simulink model "Micro_mouse"  (R2024b)
settings: Solver=FixedStepAuto  StartTime=0.0  StopTime=inf  FixedStep=0.01  RelTol=1e-3  EnableMultiTasking=on
undefined symbols (not defined in the file): DiscIntNeverNeededParam
libraries: stm32f4xxblockslib x7, simulink x4, stm32l4xxblockslib x4, slpidlib x2
settings Model: STM32="{\"PWMOutput\":[{\"ID\":\"untitled1:1\"},{\"ID\":\"Micro_mouse:1\"},{\"ID\":\"Micro_mouse:135\"},{\"ID\":\"Micro_mouse:163\"}],\"DigitalPortWrite\":[{\"ID\":\"untitled1:2\"},{\"ID\":\"Micro_mouse:2\"},{\"ID\":\"Micro_mouse:133\"},{\"ID\":\"Micro_mouse:161\"}],\"AnalogInput\":{\"ID\":\"Micro_mouse:28\"},\"DigitalPortRead\":[{\"ID\":\"Micro_mouse:101\"},{\"ID\":\"Micro_mouse:116\"},{\"ID\":\"Micro_mouse:141\"},{\"ID\":\"Micro_mouse:142\"},{\"ID\":\"Micro_mouse:169\"},{\"ID\":\"Micro_mouse:170\"}],\"HardwareInterrupt\":[{\"ID\":\"Micro_mouse:132\"},{\"ID\":\"Micro_mouse:160\"}]}"  Creator=galgi  LastModifiedBy=galgi
settings SolverCC: AutoInsertRateTranBlk=on
settings OptimizationCC: DefaultParameterBehavior=Inlined  EnhancedBackFolding=on  PassReuseOutputArgsAs=Individual arguments  ZeroExternalMemoryAtStartup=off  ZeroInternalMemoryAtStartup=off  MaxStackSize=512  OptimizeBlockOrder=speed  DifferentSizesBufferReuse=on  EfficientTunableParamExpr=on
settings DebuggingCC: ParameterTunabilityLossMsg=error
settings HardwareCC: ProdBitPerPointer=32  ProdBitPerSizeT=32  ProdBitPerPtrDiffT=32  ProdLargestAtomicInteger=Long  ProdLargestAtomicFloat=Double  ProdWordSize=32  ProdLongLongMode=on  ProdHWDeviceType=ARM Compatible->ARM Cortex-M
settings SFSimCC: MATLABDynamicMemAlloc=off
settings RTWCC: Description=Embedded Coder  SystemTargetFile=ert.tlc  HardwareBoard=STM32L4xx Based  TemplateMakefile=ert_default_tmf  Toolchain=GNU Tools for ARM Embedded Processors
settings CodeAppCC: ForceParamTrailComments=on  IgnoreCustomStorageClasses=off  OperatorAnnotations=on  SimulinkDataObjDesc=on  SFDataObjDesc=on  InsertBlockDesc=on
settings ERTTargetCC: TargetLangStandard=C99 (ISO)  CodeReplacementLibrary=ARM Cortex-M  SupportContinuousTime=on  ExtModeTransport=3  ExtModeStaticAlloc=on  ExtModeStaticAllocSize=2048  ExtModeMexFile=ext_xcp  ExtModeIntrfLevel=Level2 - Open

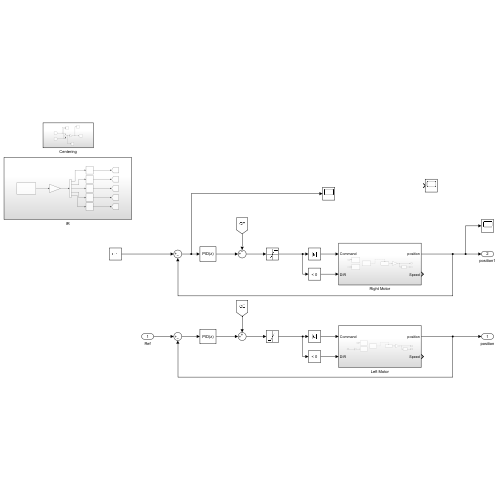
[thumbnail: Simulink's stored preview of the top-level diagram]
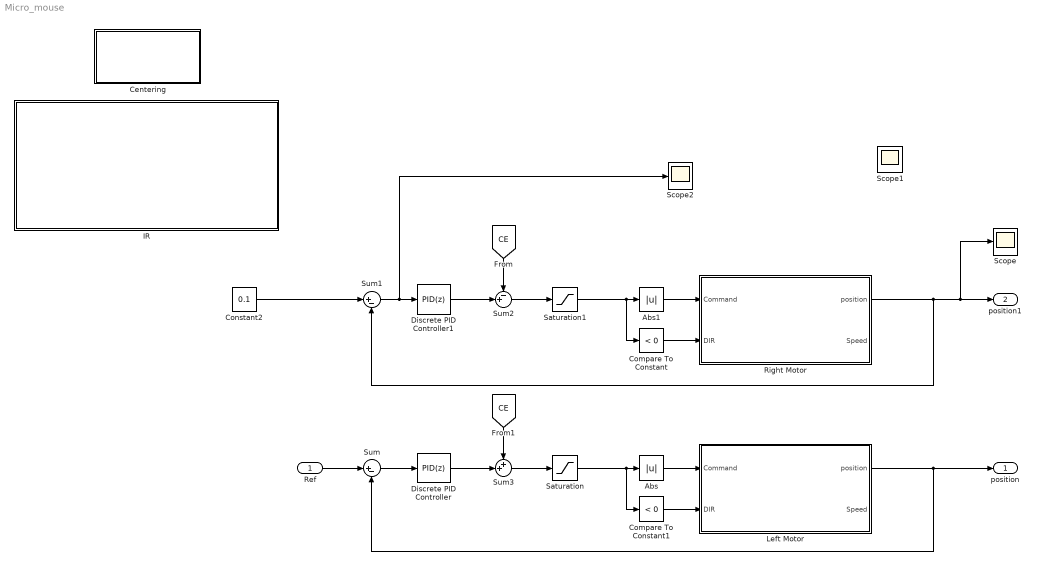
== system Micro_mouse ==
  Ref : Inport
  Abs : Abs  SaturateOnIntegerOverflow=off
  Abs1 : Abs  SaturateOnIntegerOverflow=off
  Centering : Subsystem
  Compare To Constant : simulink/Logic and Bit Operations/Compare To Constant  relop=<  const=0  OutDataTypeStr=boolean
  Compare To Constant1 : simulink/Logic and Bit Operations/Compare To Constant  relop=<  const=0  OutDataTypeStr=boolean
  Constant2 : Constant  Value=0.1
  Discrete PID Controller : slpidlib/PID Controller  Controller=PID  Form=Parallel  TimeDomain=Discrete-time  UseExternalTs=off  SampleTime=-1  IntegratorMethod=Forward Euler  FilterMethod=Forward Euler  ControllerParametersSource=internal  P=1  I=1  UseKiTs=off  D=0  UseExternalDerivativeSource=off  N=100  UseFilter=on  TunerSelectOption=Transfer Function Based (PID Tuner App)  InitialConditionSource=internal  InitialConditionForIntegrator=0  InitialConditionForFilter=0  DifferentiatorICPrevScaledInput=0  ExternalReset=none  TrackingMode=off  Kt=1  LimitOutput=off  SatLimitsSource=internal  UpperSaturationLimit=inf  LowerSaturationLimit=-inf  LinearizeAsGain=off  AntiWindupMode=none  Kb=1  LimitIntegrator=off  UpperIntegratorSaturationLimit=inf  LowerIntegratorSaturationLimit=-inf  POutMin=[]  POutMax=[]  IOutMin=[]  IOutMax=[]  DOutMin=[]  DOutMax=[]  NOutMin=[]  NOutMax=[]  SumOutMin=[]  SumOutMax=[]  SaturationOutMin=[]  SaturationOutMax=[]  PParamMin=[]  PParamMax=[]  IParamMin=[]  IParamMax=[]  DParamMin=[]  DParamMax=[]  NParamMin=[]  NParamMax=[]  KbParamMin=[]  KbParamMax=[]  KtParamMin=[]  KtParamMax=[]  KbOutMin=[]  KbOutMax=[]  KtOutMin=[]  KtOutMax=[]  IntegratorOutMin=[]  IntegratorOutMax=[]  FilterOutMin=[]  FilterOutMax=[]  SumI1OutMin=[]  SumI1OutMax=[]  SumI2OutMin=[]  SumI2OutMax=[]  SumI3OutMin=[]  SumI3OutMax=[]  SumI4OutMin=[]  SumI4OutMax=[]  SumDOutMin=[]  SumDOutMax=[]  DifferentiatorOutMin=[]  DifferentiatorOutMax=[]  FilterDiffOutCoefMin=[]  FilterDiffOutCoefMax=[]  ReciprocalOutMin=[]  ReciprocalOutMax=[]  SumDenOutMin=[]  SumDenOutMax=[]  SumNumOutMin=[]  SumNumOutMax=[]  DivideOutMin=[]  DivideOutMax=[]  UdiffTsProdOutMin=[]  UdiffTsProdOutMax=[]  NTsProdOutMin=[]  NTsProdOutMax=[]  UintegralTsProdOutMin=[]  UintegralTsProdOutMax=[]  UngainTsProdOutMin=[]  UngainTsProdOutMax=[]  ClampingZeroOutDataTypeStr=Inherit: Inherit via back propagation  ClampingZeroOutMin=[]  ClampingZeroOutMax=[]  FilterDenConstantOutDataTypeStr=Inherit: Inherit via back propagation  FilterDenConstantOutMin=[]  FilterDenConstantOutMax=[]  PCopyOutDataTypeStr=Inherit: Inherit via back propagation  PCopyOutMin=[]  PCopyOutMax=[]  NCopyOutDataTypeStr=Inherit: Inherit via back propagation  NCopyOutMin=[]  NCopyOutMax=[]  IntegratorContinuousStateAttributes=''  IntegratorStateMustResolveToSignalObject=off  IntegratorRTWStateStorageClass=Auto  FilterContinuousStateAttributes=''  FilterStateMustResolveToSignalObject=off  FilterRTWStateStorageClass=Auto  ParallelPVariant=InternalParameters  IdealPVariant=Disabled  IVariant=InternalParameters  DVariant=InternalParameters  IntegratorVariant=Discrete  SatVariant=Disabled  AWVariant=Passthrough  PCopyVariant=Disabled  TRVariant=Disabled  FdbkBlocksVariant=Forward  IdealPFdbkVariant=Disabled  SatFdbkVariant=Disabled  DerivativeFilterVariant=ForwardEulerFilter  NVariant=InternalParameters  NCopyVariant=Disabled  FilterICVariant=InternalICsFilter  IntegratorICVariant=InternalICs  ExternalResetVariant=Disabled  TRSumVariant=Passthrough  SumFdbkVariant=Disabled  SumVariant=Sum_PID  TsampFilterVariant=InternalTs  TsampNgainVariant=Passthrough  TsampIntegralVariant=Disabled_SignalSpec  ExternalSaturationOutDataTypeStr=Inherit: Same as second input  DerivativeSourceVariant=ErrorSignal  PreIntVariant=InternalPreInt
      settings: LibrarySourceBlock=simulink/Discrete/Discrete PID Controller
  Discrete PID Controller1 : slpidlib/PID Controller  Controller=PID  Form=Parallel  TimeDomain=Discrete-time  UseExternalTs=off  SampleTime=-1  IntegratorMethod=Forward Euler  FilterMethod=Forward Euler  ControllerParametersSource=internal  P=1  I=1  UseKiTs=off  D=0  UseExternalDerivativeSource=off  N=100  UseFilter=on  TunerSelectOption=Transfer Function Based (PID Tuner App)  InitialConditionSource=internal  InitialConditionForIntegrator=0  InitialConditionForFilter=0  DifferentiatorICPrevScaledInput=0  ExternalReset=none  TrackingMode=off  Kt=1  LimitOutput=off  SatLimitsSource=internal  UpperSaturationLimit=inf  LowerSaturationLimit=-inf  LinearizeAsGain=off  AntiWindupMode=none  Kb=1  LimitIntegrator=off  UpperIntegratorSaturationLimit=inf  LowerIntegratorSaturationLimit=-inf  POutMin=[]  POutMax=[]  IOutMin=[]  IOutMax=[]  DOutMin=[]  DOutMax=[]  NOutMin=[]  NOutMax=[]  SumOutMin=[]  SumOutMax=[]  SaturationOutMin=[]  SaturationOutMax=[]  PParamMin=[]  PParamMax=[]  IParamMin=[]  IParamMax=[]  DParamMin=[]  DParamMax=[]  NParamMin=[]  NParamMax=[]  KbParamMin=[]  KbParamMax=[]  KtParamMin=[]  KtParamMax=[]  KbOutMin=[]  KbOutMax=[]  KtOutMin=[]  KtOutMax=[]  IntegratorOutMin=[]  IntegratorOutMax=[]  FilterOutMin=[]  FilterOutMax=[]  SumI1OutMin=[]  SumI1OutMax=[]  SumI2OutMin=[]  SumI2OutMax=[]  SumI3OutMin=[]  SumI3OutMax=[]  SumI4OutMin=[]  SumI4OutMax=[]  SumDOutMin=[]  SumDOutMax=[]  DifferentiatorOutMin=[]  DifferentiatorOutMax=[]  FilterDiffOutCoefMin=[]  FilterDiffOutCoefMax=[]  ReciprocalOutMin=[]  ReciprocalOutMax=[]  SumDenOutMin=[]  SumDenOutMax=[]  SumNumOutMin=[]  SumNumOutMax=[]  DivideOutMin=[]  DivideOutMax=[]  UdiffTsProdOutMin=[]  UdiffTsProdOutMax=[]  NTsProdOutMin=[]  NTsProdOutMax=[]  UintegralTsProdOutMin=[]  UintegralTsProdOutMax=[]  UngainTsProdOutMin=[]  UngainTsProdOutMax=[]  ClampingZeroOutDataTypeStr=Inherit: Inherit via back propagation  ClampingZeroOutMin=[]  ClampingZeroOutMax=[]  FilterDenConstantOutDataTypeStr=Inherit: Inherit via back propagation  FilterDenConstantOutMin=[]  FilterDenConstantOutMax=[]  PCopyOutDataTypeStr=Inherit: Inherit via back propagation  PCopyOutMin=[]  PCopyOutMax=[]  NCopyOutDataTypeStr=Inherit: Inherit via back propagation  NCopyOutMin=[]  NCopyOutMax=[]  IntegratorContinuousStateAttributes=''  IntegratorStateMustResolveToSignalObject=off  IntegratorRTWStateStorageClass=Auto  FilterContinuousStateAttributes=''  FilterStateMustResolveToSignalObject=off  FilterRTWStateStorageClass=Auto  ParallelPVariant=InternalParameters  IdealPVariant=Disabled  IVariant=InternalParameters  DVariant=InternalParameters  IntegratorVariant=Discrete  SatVariant=Disabled  AWVariant=Passthrough  PCopyVariant=Disabled  TRVariant=Disabled  FdbkBlocksVariant=Forward  IdealPFdbkVariant=Disabled  SatFdbkVariant=Disabled  DerivativeFilterVariant=ForwardEulerFilter  NVariant=InternalParameters  NCopyVariant=Disabled  FilterICVariant=InternalICsFilter  IntegratorICVariant=InternalICs  ExternalResetVariant=Disabled  TRSumVariant=Passthrough  SumFdbkVariant=Disabled  SumVariant=Sum_PID  TsampFilterVariant=InternalTs  TsampNgainVariant=Passthrough  TsampIntegralVariant=Disabled_SignalSpec  ExternalSaturationOutDataTypeStr=Inherit: Same as second input  DerivativeSourceVariant=ErrorSignal  PreIntVariant=InternalPreInt
      settings: LibrarySourceBlock=simulink/Discrete/Discrete PID Controller
  IR : Subsystem
  Left Motor : Subsystem
  Right Motor : Subsystem
  Saturation : Saturate  UpperLimit=100  LowerLimit=0
  Saturation1 : Saturate  UpperLimit=100  LowerLimit=0
  Scope : Scope
  Scope1 : Scope
  Scope2 : Scope
  Sum : Sum  Inputs=|+-
  Sum1 : Sum  Inputs=|+-
  Sum2 : Sum  Inputs=-+|
  Sum3 : Sum  Inputs=++|
  position : Outport
  position1 : Outport  Port=2
  wires:
  Saturation/1 -> Compare To Constant1/1, Abs/1
  Ref/1 -> Sum/1
  Sum/1 -> Discrete PID Controller/1
  Left Motor/1(position) -> Sum/2, position/1
  Saturation1/1 -> Compare To Constant/1, Abs1/1
  Right Motor/1(position) -> Sum1/2, Scope/1, position1/1
  Sum1/1 -> Scope2/1, Discrete PID Controller1/1
  Discrete PID Controller1/1 -> Sum2/2
  Sum2/1 -> Saturation1/1
  [CE] -> Sum2/1
  [CE] -> Sum3/1
  Sum3/1 -> Saturation/1
  Discrete PID Controller/1 -> Sum3/2
  Compare To Constant/1 -> Right Motor/2(DIR)
  Compare To Constant1/1 -> Left Motor/2(DIR)
  Abs/1 -> Left Motor/1(Command)
  Abs1/1 -> Right Motor/1(Command)
  Constant2/1 -> Sum1/1

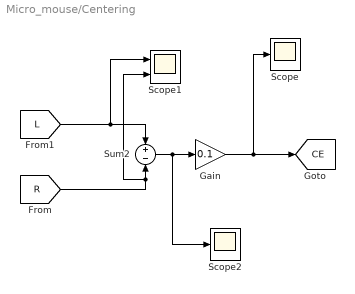
== system Micro_mouse/Centering ==
  Gain : Gain  Gain=0.1
  Scope : Scope
  Scope1 : Scope  NumInputPorts=2
  Scope2 : Scope
  Sum2 : Sum  Inputs=+|-
  tag scope: CE=global
  wires:
  [R] -> Scope1/2, Sum2/2
  [L] -> Scope1/1, Sum2/1
  Sum2/1 -> Scope2/1, Gain/1
  Gain/1 -> Scope/1, [CE]

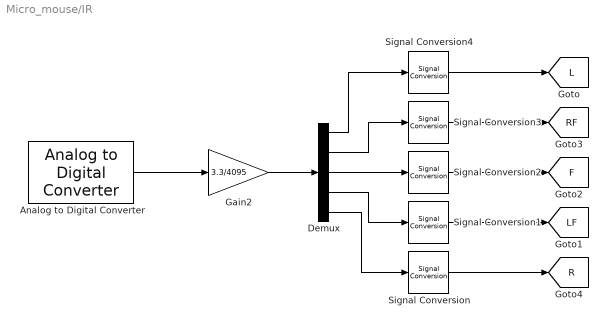
== system Micro_mouse/IR ==
  Analog to Digital Converter : stm32f4xxblockslib/Analog to Digital Converter  ADCModule=ADC1  ConversionGroup=Regular  TriggerMode=Trigger and read  NumberOfConversions=5  EnableBufferConv=off  BufferLength=1  OutputStatus=off  SampleTime=-1  EnableSimPort=off  hoistedMaskSrc=ECSoC/ECSimCodegen/Analog to Digital Converter
      settings: LibrarySourceBlock=stm32l4xxblockslib/Analog to Digital Converter
  Demux : Demux  Outputs=5
  Gain2 : Gain  Gain=3.3/4095
  Signal Conversion{,1..4} (5 alike) : SignalConversion  OverrideOpt=off
  tag scope: F=global, L=global, LF=global, R=global, RF=global
  wires:
  Demux/3 -> Signal Conversion2/1
  Demux/5 -> Signal Conversion/1
  Demux/4 -> Signal Conversion1/1
  Signal Conversion3/1 -> [RF]
  Analog to Digital Converter/1 -> Gain2/1
  Gain2/1 -> Demux/1
  Demux/2 -> Signal Conversion3/1
  Demux/1 -> Signal Conversion4/1
  Signal Conversion2/1 -> [F]
  Signal Conversion/1 -> [R]
  Signal Conversion1/1 -> [LF]
  Signal Conversion4/1 -> [L]

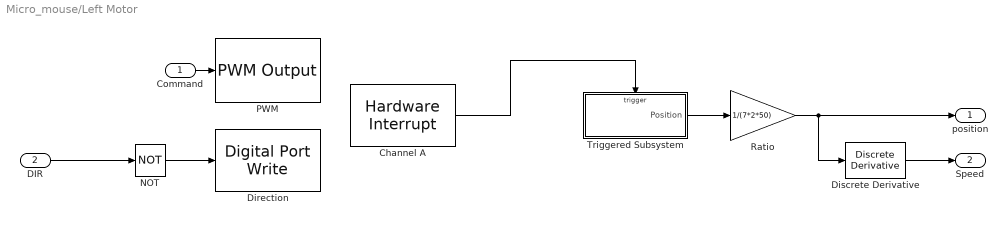
== system Micro_mouse/Left Motor ==
  Command : Inport
  DIR : Inport  Port=2
  Channel A : stm32l4xxblockslib/Hardware Interrupt  ISRGroup=External interrupts (EXTI)  ISRName=EXTI3_IRQHandler  ISRNumber=24  EventsList={ 'on', 'EXTI3 Event', '1'; 'off', 'Custom event', '2' }  SelectedEvents={'EXTI3 Event'}  TaskPriority=30  DisablePreemption=off  ClearInterruptFlagsAtEndOfEvent=off  InterruptDefinitionFile=$(TARGET_ROOT)/registry/interrupts/STM32F4xxBased_interrupts.xml  HardwareBoard=STM32L4xx Based  EnableSimPort=off
  Direction : stm32f4xxblockslib/Digital Port Write  PortName=GPIOA  PinNumber=[12]  ReadOperation=off  IOAsArray=on  EnableSimPort=off  hoistedMaskSrc=ECSoC/ECSimCodegen/Digital Port Write
      settings: LibrarySourceBlock=stm32l4xxblockslib/Digital Port Write
  Discrete Derivative : simulink/Discrete/Discrete Derivative  gainval=1.0  ICPrevScaledInput=0.0  OutMin=[]  OutMax=[]  OutDataType=fixdt(1, 16)  OutScaling=2^-10  DoSatur=off
  NOT : Logic  Operator=NOT  IconShape=distinctive  AllPortsSameDT=off
  PWM : stm32l4xxblockslib/PWM Output  TimerModule=TIM16  DutycycleUnits=Percentage  EnableChannel1=on  EnableChannel2=off  EnableChannel3=off  EnableChannel4=off  EnableChannel5=off  EnableChannel6=off  EnableCounterInput=off  EnableMainOutputInput=off  EnableFrequencyInput=off  SetRCAfterCE=off  OutputDirection=off  OutputMainOutputEnableStatus=off  SampleTime=0.1  EnableSimPort=off  EnableUpdateEvent=off  EnableCaptureCompare1Event=off  EnableCaptureCompare2Event=off  EnableCaptureCompare3Event=off  EnableCaptureCompare4Event=off  EnableTriggerEvent=off  EnableBreakEvent=off  EnableBreakEvent2=off  ProcessorFamily=STM32L4  hoistedMaskSrc=ECSoC/ECSimCodegen/PWM Output
  Ratio : Gain  Gain=1/(7*2*50)
  Triggered Subsystem : Subsystem  TreatAsAtomicUnit=on
  position : Outport
  Speed : Outport  Port=2
  wires:
  Command/1 -> PWM/1
  DIR/1 -> NOT/1
  Triggered Subsystem/1(Position) -> Ratio/1
  Channel A/1 -> Triggered Subsystem/Trigger
  Discrete Derivative/1 -> Speed/1
  Ratio/1 -> position/1, Discrete Derivative/1
  NOT/1 -> Direction/1

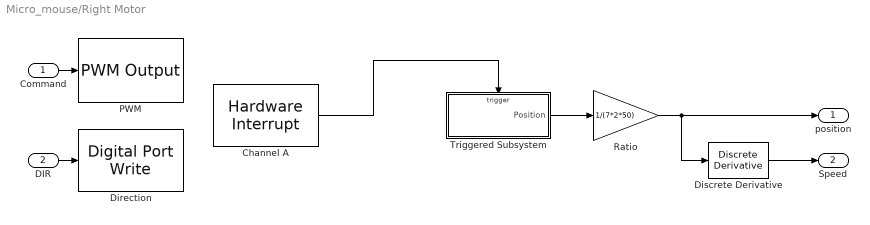
== system Micro_mouse/Right Motor ==
  Command : Inport
  DIR : Inport  Port=2
  Channel A : stm32l4xxblockslib/Hardware Interrupt  ISRGroup=External interrupts (EXTI)  ISRName=EXTI0_IRQHandler  ISRNumber=21  EventsList={ 'on', 'EXTI0 Event', '1'; 'off', 'Custom event', '2' }  SelectedEvents={'EXTI0 Event'}  TaskPriority=30  DisablePreemption=off  ClearInterruptFlagsAtEndOfEvent=off  InterruptDefinitionFile=$(TARGET_ROOT)/registry/interrupts/STM32F4xxBased_interrupts.xml  HardwareBoard=STM32L4xx Based  EnableSimPort=off
  Direction : stm32f4xxblockslib/Digital Port Write  PortName=GPIOA  PinNumber=[11]  ReadOperation=off  IOAsArray=on  EnableSimPort=off  hoistedMaskSrc=ECSoC/ECSimCodegen/Digital Port Write
      settings: LibrarySourceBlock=stm32l4xxblockslib/Digital Port Write
  Discrete Derivative : simulink/Discrete/Discrete Derivative  gainval=1.0  ICPrevScaledInput=0.0  OutMin=[]  OutMax=[]  OutDataType=fixdt(1, 16)  OutScaling=2^-10  DoSatur=off
  PWM : stm32l4xxblockslib/PWM Output  TimerModule=TIM1  DutycycleUnits=Percentage  EnableChannel1=on  EnableChannel2=off  EnableChannel3=off  EnableChannel4=off  EnableChannel5=off  EnableChannel6=off  EnableCounterInput=off  EnableMainOutputInput=off  EnableFrequencyInput=off  SetRCAfterCE=off  OutputDirection=off  OutputMainOutputEnableStatus=off  SampleTime=0.1  EnableSimPort=off  EnableUpdateEvent=off  EnableCaptureCompare1Event=off  EnableCaptureCompare2Event=off  EnableCaptureCompare3Event=off  EnableCaptureCompare4Event=off  EnableTriggerEvent=off  EnableBreakEvent=off  EnableBreakEvent2=off  ProcessorFamily=STM32L4  hoistedMaskSrc=ECSoC/ECSimCodegen/PWM Output
  Ratio : Gain  Gain=1/(7*2*50)
  Triggered Subsystem : Subsystem  TreatAsAtomicUnit=on
  position : Outport
  Speed : Outport  Port=2
  wires:
  Command/1 -> PWM/1
  DIR/1 -> Direction/1
  Triggered Subsystem/1(Position) -> Ratio/1
  Channel A/1 -> Triggered Subsystem/Trigger
  Discrete Derivative/1 -> Speed/1
  Ratio/1 -> position/1, Discrete Derivative/1

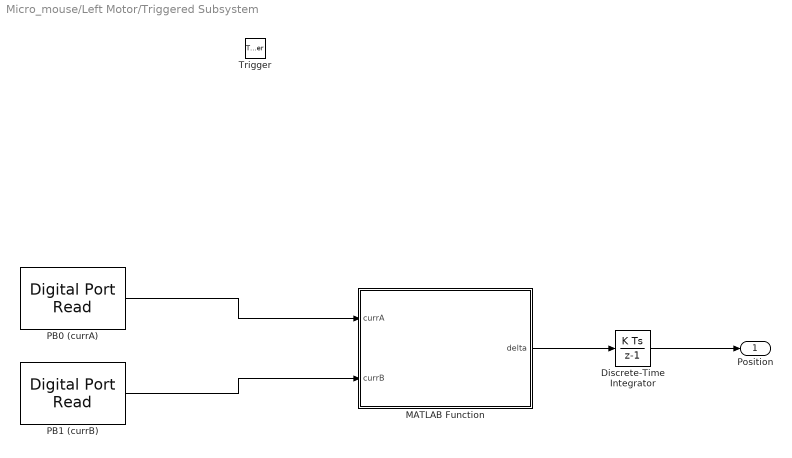
== system Micro_mouse/Left Motor/Triggered Subsystem ==
  Trigger : TriggerPort  TriggerType=function-call  VariantControl=(inherit)
  Discrete-Time Integrator : DiscreteIntegrator  SampleTime=-1  ICPrevOutput=DiscIntNeverNeededParam  ICPrevScaledInput=DiscIntNeverNeededParam
  MATLAB Function : MATLAB Function  TreatAsAtomicUnit=on
  PB0 (currA) : stm32f4xxblockslib/Digital Port Read  PortName=GPIOB  PinNumber=[3]  ReadOperation=on  IOAsArray=on  SampleTime=-1  EnableSimPort=off  hoistedMaskSrc=ECSoC/ECSimCodegen/Digital Port Read
      settings: LibrarySourceBlock=stm32l4xxblockslib/Digital Port Read
  PB1 (currB) : stm32f4xxblockslib/Digital Port Read  PortName=GPIOB  PinNumber=[4]  ReadOperation=on  IOAsArray=on  SampleTime=-1  EnableSimPort=off  hoistedMaskSrc=ECSoC/ECSimCodegen/Digital Port Read
      settings: LibrarySourceBlock=stm32l4xxblockslib/Digital Port Read
  Position : Outport
  wires:
  PB1 (currB)/1 -> MATLAB Function/2(currB)
  PB0 (currA)/1 -> MATLAB Function/1(currA)
  Discrete-Time Integrator/1 -> Position/1
  MATLAB Function/1(delta) -> Discrete-Time Integrator/1

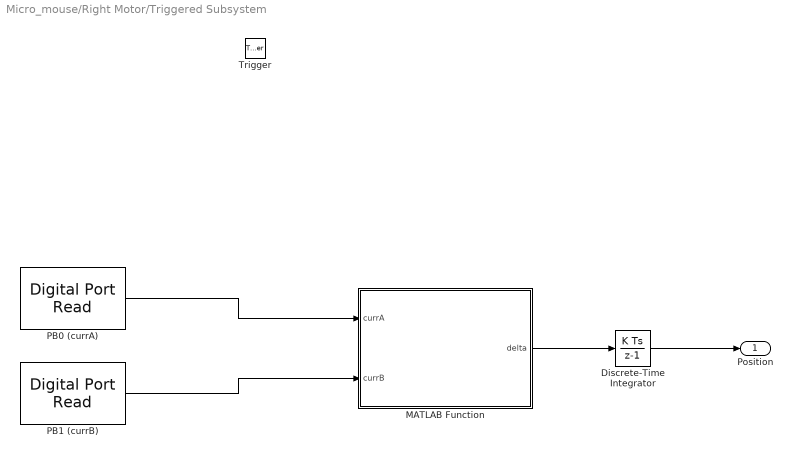
== system Micro_mouse/Right Motor/Triggered Subsystem ==
  Trigger : TriggerPort  TriggerType=function-call  VariantControl=(inherit)
  Discrete-Time Integrator : DiscreteIntegrator  SampleTime=-1  ICPrevOutput=DiscIntNeverNeededParam  ICPrevScaledInput=DiscIntNeverNeededParam
  MATLAB Function : MATLAB Function  TreatAsAtomicUnit=on
  PB0 (currA) : stm32f4xxblockslib/Digital Port Read  PortName=GPIOB  PinNumber=[0]  ReadOperation=on  IOAsArray=on  SampleTime=-1  EnableSimPort=off  hoistedMaskSrc=ECSoC/ECSimCodegen/Digital Port Read
      settings: LibrarySourceBlock=stm32l4xxblockslib/Digital Port Read
  PB1 (currB) : stm32f4xxblockslib/Digital Port Read  PortName=GPIOB  PinNumber=[1]  ReadOperation=on  IOAsArray=on  SampleTime=-1  EnableSimPort=off  hoistedMaskSrc=ECSoC/ECSimCodegen/Digital Port Read
      settings: LibrarySourceBlock=stm32l4xxblockslib/Digital Port Read
  Position : Outport
  wires:
  PB1 (currB)/1 -> MATLAB Function/2(currB)
  PB0 (currA)/1 -> MATLAB Function/1(currA)
  Discrete-Time Integrator/1 -> Position/1
  MATLAB Function/1(delta) -> Discrete-Time Integrator/1

== matlab function Micro_mouse/Left Motor/Triggered Subsystem/MATLAB Function ==
  data: delta output; currA input; currB input
function delta = decodeSimple(currA, currB)
    if (currA == currB)
        delta = +1;   % Forward
    else
        delta = -1;   % Reverse
    end
end

== matlab function Micro_mouse/Right Motor/Triggered Subsystem/MATLAB Function ==
  data: delta output; currA input; currB input
function delta = decodeSimple(currA, currB)
    if (currA == currB)
        delta = -1;   % Forward
    else
        delta = +1;   % Reverse
    end
end
